simulink model "dos_attack"  (R2021a)
settings: Solver=VariableStepAuto  StartTime=0.0  StopTime=10.0  RelTol=1e-3
values from neighbouring files (symbols this model uses):
  probability = 2^(-4)    (= 0.0625)    [attack_setUp.m]
settings Model: Creator=uidk9388  LastModifiedBy=uidk9388

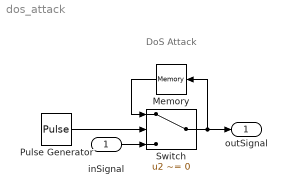
== system dos_attack ==
  note: DoS Attack
  inSignal : Inport
  Memory : Memory
  Pulse Generator : DiscretePulseGenerator  PulseType=Time based  Period=1  PulseWidth=90
  Switch : Switch  Criteria=u2 ~= 0  Threshold=probability
  outSignal : Outport
  wires:
  Memory/1 -> Switch/1
  Switch/1 -> Memory/1, outSignal/1
  Pulse Generator/1 -> Switch/2
  inSignal/1 -> Switch/3
